simulink model "The_SIMULINK_robot_model"  (R2016b)
settings: Solver=VariableStepAuto  StartTime=0.0  StopTime=20  RelTol=1e-3
undefined symbols (not defined in the file): g, L, m, mu, mu1, mu2, tou1, wn
settings Model: Creator=Administrator  LastModifiedBy=Administrator
settings DebuggingCC: SFMachineParentedDataDiag=error
settings SFSimCC: SimUseLocalCustomCode=on
settings RTWCC: RTWUseLocalCustomCode=on

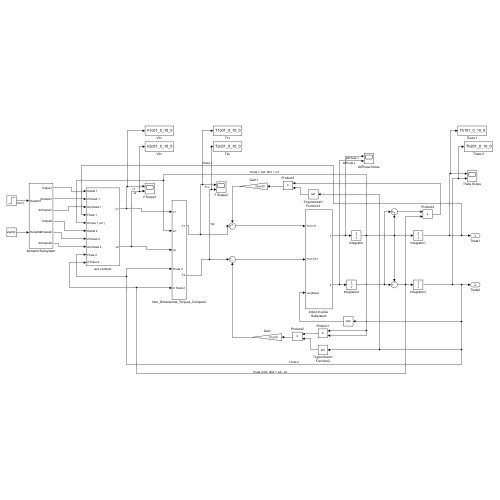
[thumbnail: Simulink's stored preview of the top-level diagram]
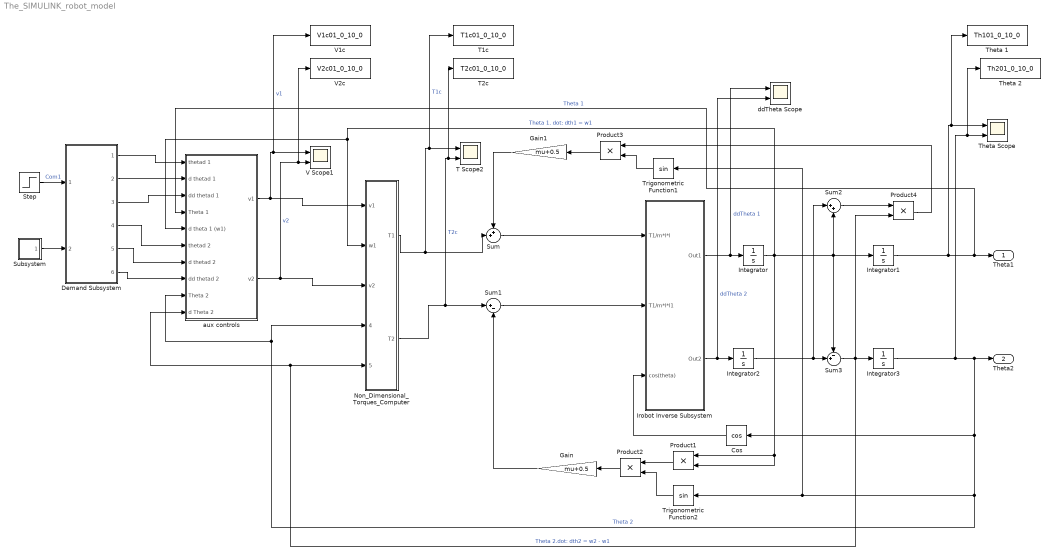
== system The_SIMULINK_robot_model ==
  Cos : Trigonometry  Operator=cos
  Demand Subsystem : Subsystem
  Gain : Gain  Gain=mu+0.5
  Gain1 : Gain  Gain=mu+0.5
  Integrator{,1..3} (4 alike) : Integrator
  Irobot Inverse Subsystem : Subsystem
  Non_Dimensional_Torques_Computer : Subsystem
  Product{1..4} (4 alike) : Product
  Step : Step  After=6.87*pi/180  SampleTime=0
  Subsystem : Subsystem
  Sum : Sum  Inputs=++|
  Sum1 : Sum  Inputs=|+-
  Sum2 : Sum  Inputs=|++
  Sum3 : Sum  Inputs=-+|
  T Scope2 : Scope  NumInputPorts=2
  T1c : ToWorkspace  VariableName=T1c01_0_10_0  SaveFormat=Timeseries  SampleTime=-1
  T2c : ToWorkspace  VariableName=T2c01_0_10_0  SaveFormat=Timeseries  SampleTime=-1
  Theta 1 : ToWorkspace  VariableName=Th101_0_10_0  SaveFormat=Timeseries  SampleTime=-1
  Theta 2 : ToWorkspace  VariableName=Th201_0_10_0  SaveFormat=Timeseries  SampleTime=-1
  Theta Scope : Scope  NumInputPorts=2
  Trigonometric Function1 : Trigonometry
  Trigonometric Function2 : Trigonometry
  V Scope1 : Scope  NumInputPorts=2
  V1c : ToWorkspace  VariableName=V1c01_0_10_0  SaveFormat=Timeseries  SampleTime=-1
  V2c : ToWorkspace  VariableName=V2c01_0_10_0  SaveFormat=Timeseries  SampleTime=-1
  aux controls : Subsystem
  ddTheta Scope : Scope  NumInputPorts=2
  Theta1 : Outport
  Theta2 : Outport  Port=2
  wires:
  Non_Dimensional_Torques_Computer/1(T1) -> T1c/1, T Scope2/1, Sum/2  "T1c"
  Gain1/1 -> Sum/1
  Sum1/1 -> Irobot Inverse Subsystem/2(T1/m*l*l1)
  Sum/1 -> Irobot Inverse Subsystem/1(T1/m*l*l)
  Product3/1 -> Gain1/1
  Trigonometric Function1/1 -> Product3/2
  Gain/1 -> Sum1/2
  Product2/1 -> Gain/1
  Product1/1 -> Product2/1
  Trigonometric Function2/1 -> Product2/2
  Cos/1 -> Irobot Inverse Subsystem/3(cos(theta))
  Irobot Inverse Subsystem/2(Out2) -> ddTheta Scope/2, Integrator2/1  "ddTheta 2"
  Integrator/1 -> Non_Dimensional_Torques_Computer/2(w1), aux controls/5(d theta 1 (w1)), Product1/2, Product1/1, Sum3/1, Sum2/2, Integrator1/1  "Theta 1. dot: dth1 = w1"
  Integrator1/1 -> Theta 1/1, Theta Scope/1, aux controls/4(Theta 1), Theta1/1  "Theta 1"
  Integrator3/1 -> Theta 2/1, Theta Scope/2, Non_Dimensional_Torques_Computer/4(Theta 2), aux controls/9(Theta 2), Trigonometric Function1/1, Trigonometric Function2/1, Cos/1, Theta2/1  "Theta 2"
  Sum2/1 -> Product4/1
  Integrator2/1 -> Sum2/1, Sum3/2
  Sum3/1 -> Non_Dimensional_Torques_Computer/5(d Theta 2 w2-w1), aux controls/10(d Theta 2), Product4/2, Integrator3/1  "Theta 2.dot: dth2 = w2 - w1"
  Product4/1 -> Product3/1
  Non_Dimensional_Torques_Computer/2(T2) -> T2c/1, T Scope2/2, Sum1/1  "T2c"
  aux controls/1(v1) -> V1c/1, V Scope1/1, Non_Dimensional_Torques_Computer/1(v1)  "v1"
  aux controls/2(v2) -> V2c/1, V Scope1/2, Non_Dimensional_Torques_Computer/3(v2)  "v2"
  Step/1 -> Demand Subsystem/1(thetad01)  "Com1"
  Demand Subsystem/1(thetad1) -> aux controls/1(thetad 1)
  Demand Subsystem/2(d thetad1) -> aux controls/2(d thetad 1)
  Demand Subsystem/3(dd thetad1) -> aux controls/3(dd thetad 1)
  Demand Subsystem/4(thetad2) -> aux controls/6(thetad 2)
  Demand Subsystem/5(d thetad2) -> aux controls/7(d thetad 2)
  Demand Subsystem/6(dd thetad2) -> aux controls/8(dd thetad 2)
  Subsystem/1(thetad02) -> Demand Subsystem/2(thetad02)
  Irobot Inverse Subsystem/1(Out1) -> ddTheta Scope/1, Integrator/1  "ddTheta 1"

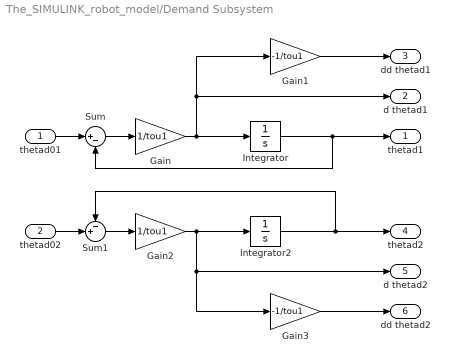
== system The_SIMULINK_robot_model/Demand Subsystem ==
  thetad01 : Inport
  thetad02 : Inport  Port=2
  Gain : Gain  Gain=1/tou1
  Gain1 : Gain  Gain=-1/tou1
  Gain2 : Gain  Gain=1/tou1
  Gain3 : Gain  Gain=-1/tou1
  Integrator : Integrator
  Integrator2 : Integrator
  Sum : Sum  Inputs=|+-
  Sum1 : Sum  Inputs=-+|
  thetad1 : Outport
  d thetad1 : Outport  Port=2
  dd thetad1 : Outport  Port=3
  thetad2 : Outport  Port=4
  d thetad2 : Outport  Port=5
  dd thetad2 : Outport  Port=6
  wires:
  Integrator/1 -> thetad1/1, Sum/2
  thetad01/1 -> Sum/1
  Sum/1 -> Gain/1
  Gain/1 -> Gain1/1, d thetad1/1, Integrator/1
  Gain1/1 -> dd thetad1/1
  Sum1/1 -> Gain2/1
  Gain2/1 -> Gain3/1, d thetad2/1, Integrator2/1
  Integrator2/1 -> thetad2/1, Sum1/1
  thetad02/1 -> Sum1/2
  Gain3/1 -> dd thetad2/1

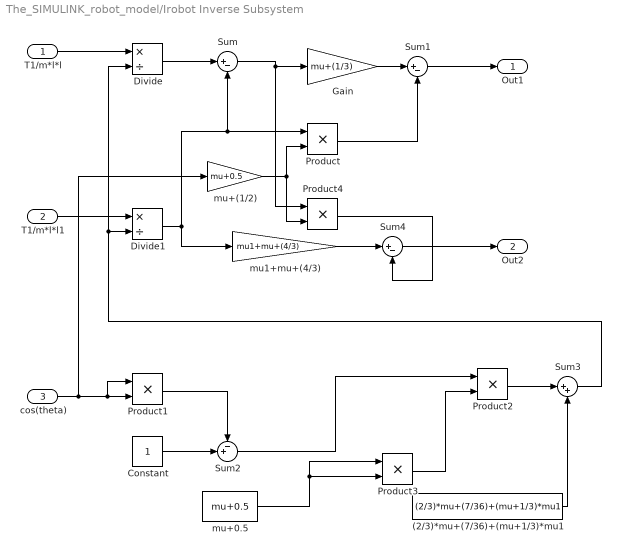
== system The_SIMULINK_robot_model/Irobot Inverse Subsystem ==
  T1/m*l*l : Inport
  T1/m*l*l1 : Inport  Port=2
  cos(theta) : Inport  Port=3
  (2/3)*mu+(7/36)+(mu+1/3)*mu1 : Constant  Value=(2/3)*mu+(7/36)+(mu+1/3)*mu1
  Constant : Constant
  Divide : Product  Inputs=*/
  Divide1 : Product  Inputs=*/
  Gain : Gain  Gain=mu+(1/3)
  Product{,1..4} (5 alike) : Product
  Sum : Sum  Inputs=|+-
  Sum1 : Sum  Inputs=|+-
  Sum2 : Sum  Inputs=-+|
  Sum3 : Sum  Inputs=|++
  Sum4 : Sum  Inputs=|+-
  mu+(1/2) : Gain  Gain=mu+0.5
  mu+0.5 : Constant  Value=mu+0.5
  mu1+mu+(4/3) : Gain  Gain=mu1+mu+(4/3)
  Out1 : Outport
  Out2 : Outport  Port=2
  wires:
  Sum4/1 -> Out2/1
  Product4/1 -> Sum4/2
  mu+0.5/1 -> Product3/2, Product3/1
  Product3/1 -> Product2/2
  Sum3/1 -> Divide1/2, Divide/2
  (2/3)*mu+(7/36)+(mu+1/3)*mu1/1 -> Sum3/2
  Divide1/1 -> mu1+mu+(4/3)/1, Sum/2, Product/1
  mu1+mu+(4/3)/1 -> Sum4/1
  Product2/1 -> Sum3/1
  Divide/1 -> Sum/1
  Sum2/1 -> Product2/1
  Sum1/1 -> Out1/1
  Product1/1 -> Sum2/1
  Constant/1 -> Sum2/2
  mu+(1/2)/1 -> Product/2, Product4/2
  cos(theta)/1 -> mu+(1/2)/1, Product1/2, Product1/1
  T1/m*l*l1/1 -> Divide1/1
  Gain/1 -> Sum1/1
  T1/m*l*l/1 -> Divide/1
  Product/1 -> Sum1/2
  Sum/1 -> Product4/1, Gain/1

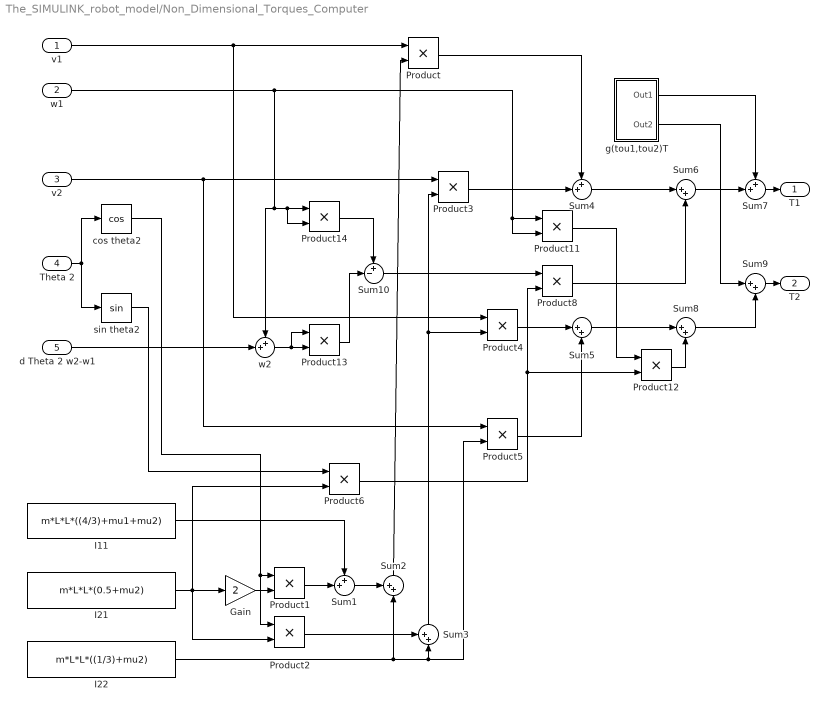
== system The_SIMULINK_robot_model/Non_Dimensional_Torques_Computer ==
  v1 : Inport
  w1 : Inport  Port=2
  v2 : Inport  Port=3
  Theta 2 : Inport  Port=4
  d Theta 2 w2-w1 : Inport  Port=5
  Gain : Gain  Gain=2
  I11 : Constant  Value=m*L*L*((4/3)+mu1+mu2)
  I21 : Constant  Value=m*L*L*(0.5+mu2)
  I22 : Constant  Value=m*L*L*((1/3)+mu2)
  Product{,1..6,8,11..14} (12 alike) : Product
  Sum{1..4,7} (5 alike) : Sum  Inputs=++|
  Sum10 : Sum  Inputs=+-|
  Sum{5..6,8..9} (4 alike) : Sum  Inputs=|++
  cos theta2 : Trigonometry  Operator=cos
  g(tou1,tou2)T : Subsystem
  sin theta2 : Trigonometry
  w2 : Sum  Inputs=++|
  T1 : Outport
  T2 : Outport  Port=2
  wires:
  v1/1 -> Product/1, Product4/1
  Sum2/1 -> Product/2
  Theta 2/1 -> cos theta2/1, sin theta2/1
  Gain/1 -> Product1/2
  I21/1 -> Product6/2, Product2/2, Gain/1
  cos theta2/1 -> Product2/1, Product1/1
  Product1/1 -> Sum1/2
  I11/1 -> Sum1/1
  Sum1/1 -> Sum2/1
  I22/1 -> Product5/2, Sum3/2, Sum2/2
  Product2/1 -> Sum3/1
  Sum3/1 -> Product4/2, Product3/2
  v2/1 -> Product3/1, Product5/1
  Product/1 -> Sum4/1
  Product3/1 -> Sum4/2
  Product4/1 -> Sum5/1
  Product5/1 -> Sum5/2
  sin theta2/1 -> Product6/1
  Product6/1 -> Product8/2, Product12/2
  w1/1 -> Product11/2, Product11/1, Product14/2, Product14/1, w2/1
  Sum4/1 -> Sum6/1
  Product8/1 -> Sum6/2
  Sum6/1 -> Sum7/2
  Sum7/1 -> T1/1
  Product11/1 -> Product12/1
  Sum5/1 -> Sum8/1
  Sum8/1 -> Sum9/2
  Sum9/1 -> T2/1
  d Theta 2 w2-w1/1 -> w2/2
  w2/1 -> Product13/1, Product13/2
  Product13/1 -> Sum10/2
  Product14/1 -> Sum10/1
  Sum10/1 -> Product8/1
  g(tou1,tou2)T/1(Out1) -> Sum7/1
  g(tou1,tou2)T/2(Out2) -> Sum9/1
  Product12/1 -> Sum8/2

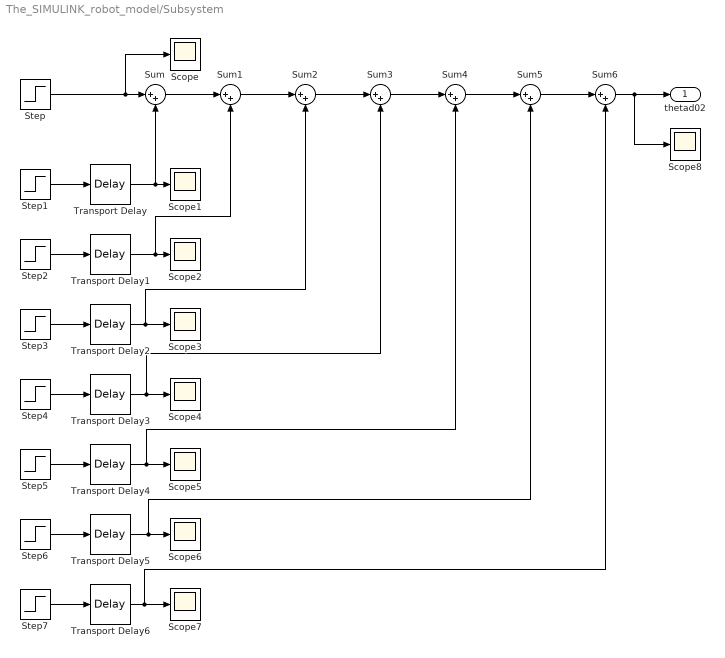
== system The_SIMULINK_robot_model/Subsystem ==
  Scope{,1..8} (9 alike) : Scope
  Step{,1..7} (8 alike) : Step  After=30*pi/180  SampleTime=0
  Sum{,1..6} (7 alike) : Sum  Inputs=|++
  Transport Delay : TransportDelay
  Transport Delay1 : TransportDelay  DelayTime=2
  Transport Delay2 : TransportDelay  DelayTime=3
  Transport Delay3 : TransportDelay  DelayTime=4
  Transport Delay4 : TransportDelay  DelayTime=5
  Transport Delay5 : TransportDelay  DelayTime=6
  Transport Delay6 : TransportDelay  DelayTime=7
  thetad02 : Outport
  wires:
  Sum6/1 -> Scope8/1, thetad02/1
  Sum2/1 -> Sum3/1
  Sum3/1 -> Sum4/1
  Sum5/1 -> Sum6/1
  Sum4/1 -> Sum5/1
  Transport Delay/1 -> Sum/2, Scope1/1
  Sum1/1 -> Sum2/1
  Step/1 -> Scope/1, Sum/1
  Sum/1 -> Sum1/1
  Step1/1 -> Transport Delay/1
  Step2/1 -> Transport Delay1/1
  Transport Delay2/1 -> Sum2/2, Scope3/1
  Step3/1 -> Transport Delay2/1
  Step4/1 -> Transport Delay3/1
  Transport Delay3/1 -> Sum3/2, Scope4/1
  Transport Delay4/1 -> Sum4/2, Scope5/1
  Step5/1 -> Transport Delay4/1
  Step6/1 -> Transport Delay5/1
  Transport Delay5/1 -> Sum5/2, Scope6/1
  Transport Delay6/1 -> Sum6/2, Scope7/1
  Step7/1 -> Transport Delay6/1
  Transport Delay1/1 -> Sum1/2, Scope2/1

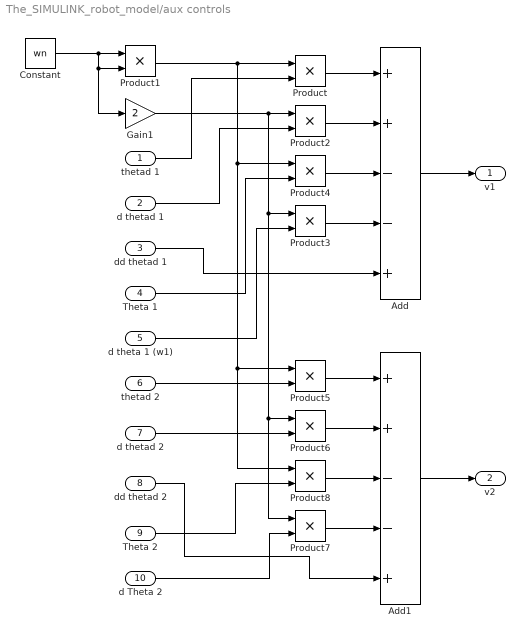
== system The_SIMULINK_robot_model/aux controls ==
  thetad 1 : Inport
  d thetad 1 : Inport  Port=2
  dd thetad 1 : Inport  Port=3
  Theta 1 : Inport  Port=4
  d theta 1 (w1) : Inport  Port=5
  thetad 2 : Inport  Port=6
  d thetad 2 : Inport  Port=7
  dd thetad 2 : Inport  Port=8
  Theta 2 : Inport  Port=9
  d Theta 2 : Inport  Port=10
  Add : Sum  Inputs=++--+
  Add1 : Sum  Inputs=++--+
  Constant : Constant  Value=wn
  Gain1 : Gain  Gain=2
  Product{,1..8} (9 alike) : Product
  v1 : Outport
  v2 : Outport  Port=2
  wires:
  Constant/1 -> Gain1/1, Product1/2, Product1/1
  Gain1/1 -> Product2/1, Product3/1, Product7/1, Product6/1
  d thetad 1/1 -> Product2/2
  Product1/1 -> Product/1, Product4/1, Product8/1, Product5/1
  thetad 1/1 -> Product/2
  d theta 1 (w1)/1 -> Product3/2
  Theta 1/1 -> Product4/2
  Product/1 -> Add/1
  Product2/1 -> Add/2
  Product4/1 -> Add/3
  Product3/1 -> Add/4
  dd thetad 1/1 -> Add/5
  thetad 2/1 -> Product5/2
  Product5/1 -> Add1/1
  d thetad 2/1 -> Product6/2
  Product8/1 -> Add1/3
  Product7/1 -> Add1/4
  d Theta 2/1 -> Product7/2
  Theta 2/1 -> Product8/2
  dd thetad 2/1 -> Add1/5
  Add/1 -> v1/1
  Add1/1 -> v2/1
  Product6/1 -> Add1/2

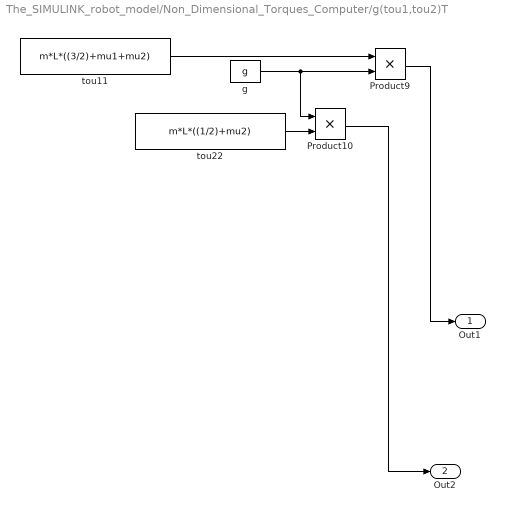
== system The_SIMULINK_robot_model/Non_Dimensional_Torques_Computer/g(tou1,tou2)T ==
  Product10 : Product
  Product9 : Product
  g : Constant  Value=g
  tou11 : Constant  Value=m*L*((3/2)+mu1+mu2)
  tou22 : Constant  Value=m*L*((1/2)+mu2)
  Out1 : Outport
  Out2 : Outport  Port=2
  wires:
  Product10/1 -> Out2/1
  Product9/1 -> Out1/1
  tou11/1 -> Product9/1
  tou22/1 -> Product10/2
  g/1 -> Product10/1, Product9/2
